simulink model "real_world_idmt_relay_3phase_standalone_2024a"  (R2024a)
settings: Solver=ode23tb  StartTime=0.0  StopTime=10  RelTol=1e-7  EnableMultiTasking=on
libraries: spsThreePhaseVIMeasurementLib x3, spsThreePhaseBreakerLib x2, spsDistributedParametersLineLib x2, spsRMSLib x2, spsThreePhaseFaultLib x2, spsThreePhaseSeriesRLCLoadLib x1, spsThreePhaseSourceLib x1, spspowerguiLib x1
settings Model: Creator=Rodney Tan  LastModifiedBy=user
settings SolverCC: AlgebraicLoopSolver=TrustRegion
settings DataIOCC: LimitDataPoints=on  SaveFormat=Array  ReturnWorkspaceOutputs=off
settings OptimizationCC: LifeSpan=inf
settings DebuggingCC: UnconnectedInputMsg=warning  UnconnectedOutputMsg=warning  UnconnectedLineMsg=warning  SFUnexpectedBacktrackingDiag=warning  SFNoUnconditionalDefaultTransitionDiag=warning  SFExecutionAtInitializationDiag=none  ArithmeticOperatorsInVariantConditions=warning
settings HardwareCC: ProdBitPerPointer=32  ProdBitPerSizeT=32  ProdBitPerPtrDiffT=32  ProdLargestAtomicFloat=None  ProdIntDivRoundTo=Undefined  ProdEndianess=Unspecified  ProdWordSize=32  ProdHWDeviceType=32-bit Generic
settings ModelReferenceCC: EnableRefExpFcnMdlSchedulingChecks=on  PropagateSignalLabelsOutOfModel=off
settings SFSimCC: SimUseLocalCustomCode=off  CustomCodeUndefinedFunction=UseInterfaceOnly
settings RTWCC: RTWUseLocalCustomCode=off  GPUComputeCapability=3.5
settings CodeAppCC: StateflowObjectComments=on
settings GRTTargetCC: TargetLangStandard=C89/C90 (ANSI)
settings ConfigComp: CovMetricSettings=dw  CovSaveCumulativeToWorkspaceVar=on  CovSaveSingleToWorkspaceVar=on  CovExternalEMLEnable=off
settings SimscapeCC: SimscapeNormalizeSystem=off

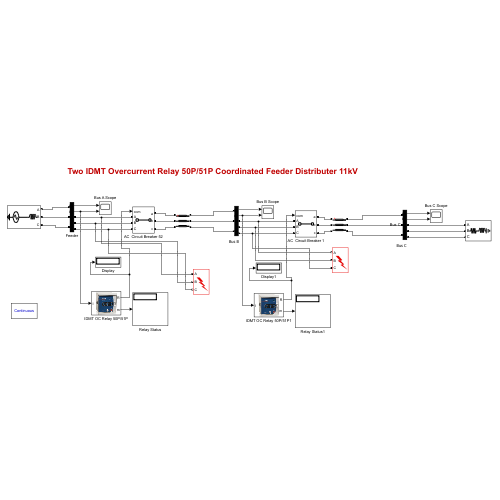
[thumbnail: Simulink's stored preview of the top-level diagram]
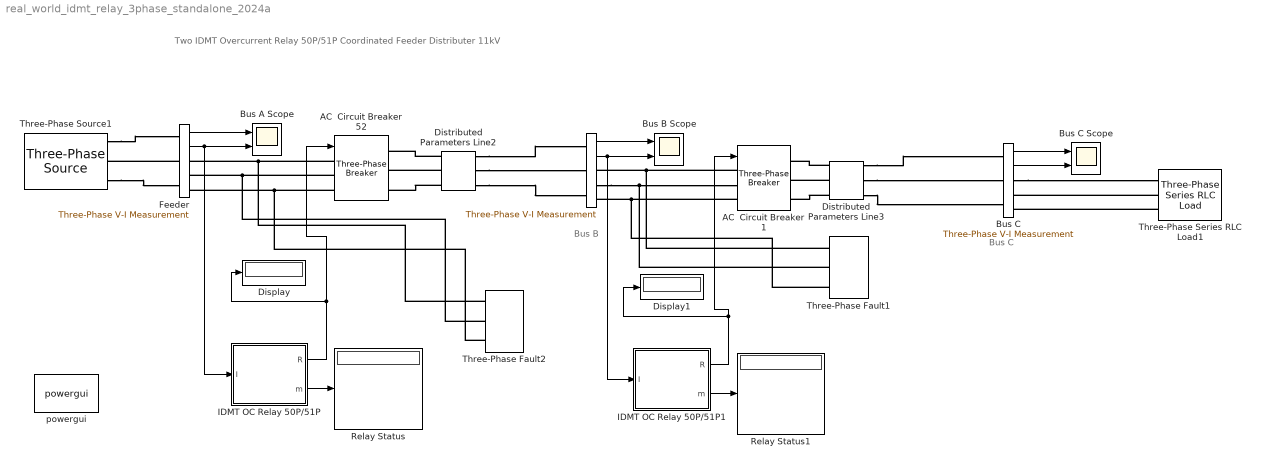
== system real_world_idmt_relay_3phase_standalone_2024a ==
  note: Bus C
  note: Bus B
  note: Two IDMT Overcurrent Relay 50P/51P Coordinated Feeder Distributer 11kV
  " " : spsThreePhaseVIMeasurementLib/Three-Phase V-I Measurement  VoltageMeasurement=phase-to-ground  SetLabelV=off  LabelV=Vabc  Vpu=off  VpuLL=off  CurrentMeasurement=yes  SetLabelI=off  LabelI=Iabc  Ipu=off  Pbase=100e6  Vbase=500e3  OutputType=Complex  PhasorSimulation=off  PSBequivalent=0
  AC  Circuit Breaker 1 : spsThreePhaseBreakerLib/Three-Phase Breaker  InitialState=closed  SwitchA=on  SwitchB=on  SwitchC=on  SwitchTimes="[1/60  5/60]"  External=on  BreakerResistance=0.01  SnubberResistance=1e6  SnubberCapacitance=inf  Measurements=None
  AC  Circuit Breaker 52 : spsThreePhaseBreakerLib/Three-Phase Breaker  InitialState=closed  SwitchA=on  SwitchB=on  SwitchC=on  SwitchTimes="[1/60  5/60]"  External=on  BreakerResistance=0.01  SnubberResistance=1e6  SnubberCapacitance=inf  Measurements=None
  Bus A Scope : Scope  NumInputPorts=2
  Bus B Scope : Scope  NumInputPorts=2
  Bus C : spsThreePhaseVIMeasurementLib/Three-Phase V-I Measurement  VoltageMeasurement=phase-to-ground  SetLabelV=off  LabelV=Vabc  Vpu=off  VpuLL=off  CurrentMeasurement=yes  SetLabelI=off  LabelI=Iabc  Ipu=off  Pbase=100e6  Vbase=500e3  OutputType=Complex  PhasorSimulation=off  PSBequivalent=0
  Bus C Scope : Scope  NumInputPorts=2
  Display : Display
  Display1 : Display
  Distributed Parameters Line2 : spsDistributedParametersLineLib/Distributed Parameters Line  Phases=3  Length=5  Frequency=50  Resistance=[0.306 0.918]  Inductance="[0.2642e-3  1.0504e-3]"  Capacitance=[12.74e-6 7.751e-6]  x1=[3.27922978200512e-12 11154.6811765329 11154.6811765329;314.159265358979 314.159265358979 314.159265358979;-1.12452839492294 0.423971778555255 -1.14682454823964]  x2=[8.7354113531085e-12 10968.40053619 10968.40053619;314.159265358979 314.159265358979 314.159265358979;-0.816475613899162 0.387208845042316 -1.18358748175258]  x3=[1.00471196056486e-12 1773.2701065899 1773.2701065899;314.159265358979 314.159265358979 314.159265358979;-1.33202462135814 0.268764817665929 -1.30203150912897]  x4=[3.36344440757806e-13 2029.84067808505 2029.84067808505;314.159265358979 314.159265358979 314.159265358979;-2.69532472171784 0.432839711669644 -1.13795661512525]  x5=0.000451155472093601  V1=[3.279e-12 1.115e+04 1.115e+04;314.2 314.2 314.2;-1.125 0.424 -1.147]  V2=[8.735e-12 1.097e+04 1.097e+04;314.2 314.2 314.2;-0.8165 0.3872 -1.184]  I1=[1.005e-12 1773 1773;314.2 314.2 314.2;-1.332 0.2688 -1.302]  I2=[3.363e-13 2030 2030;314.2 314.2 314.2;-2.695 0.4328 -1.138]  nHarmo=1  Measurements=None  Decoupling=off  VsMag0=0  VrMag0=0  VsAngle0=0  VrAngle0=0  IsMag0=0  IrMag0=0  IsAngle0=0  IrAngle0=0
      settings: LibrarySourceBlock=sps_lib/Power Grid Elements/Distributed Parameters Line
  Distributed Parameters Line3 : spsDistributedParametersLineLib/Distributed Parameters Line  Phases=3  Length=5  Frequency=50  Resistance=[0.306 0.918]  Inductance="[0.2642e-3  1.0504e-3]"  Capacitance=[12.74e-6 7.751e-6]  x1=[9.97338802310938e-12 10966.6241293561 10966.6241293561;314.159265358979 314.159265358979 314.159265358979;-0.959379717508311 0.387108931168386 -1.18368739562651]  x2=[1.28621974215375e-11 10696.5004802315 10696.5004802315;314.159265358979 314.159265358979 314.159265358979;-0.927132835073057 0.380128350784861 -1.19066797601004]  x3=[1.56443975399813e-12 1729.68176986228 1729.68176986227;314.159265358979 314.159265358979 314.159265358979;-1.2488833894697 0.333543848383118 -1.23725247841178]  x4=[1.04295983599876e-12 1982.49698055263 1982.49698055264;314.159265358979 314.159265358979 314.159265358979;-1.89238449826298 0.33489650149686 -1.23589982529804]  x5=0.000451155472093601  V1=[9.973e-12 1.097e+04 1.097e+04;314.2 314.2 314.2;-0.9594 0.3871 -1.184]  V2=[1.286e-11 1.07e+04 1.07e+04;314.2 314.2 314.2;-0.9271 0.3801 -1.191]  I1=[1.564e-12 1730 1730;314.2 314.2 314.2;-1.249 0.3335 -1.237]  I2=[1.043e-12 1982 1982;314.2 314.2 314.2;-1.892 0.3349 -1.236]  nHarmo=1  Measurements=None  Decoupling=off  VsMag0=0  VrMag0=0  VsAngle0=0  VrAngle0=0  IsMag0=0  IrMag0=0  IsAngle0=0  IrAngle0=0
      settings: LibrarySourceBlock=sps_lib/Power Grid Elements/Distributed Parameters Line
  Feeder : spsThreePhaseVIMeasurementLib/Three-Phase V-I Measurement  VoltageMeasurement=phase-to-ground  SetLabelV=off  LabelV=Vabc  Vpu=off  VpuLL=off  CurrentMeasurement=yes  SetLabelI=off  LabelI=Iabc  Ipu=off  Pbase=100e6  Vbase=500e3  OutputType=Complex  PhasorSimulation=off  PSBequivalent=0
  IDMT OC Relay 50P/51P : Subsystem  mask(IDMT Overcurrent Relay 50P/51P Block){Lowset_idx=5, TMS_idx=0.2, Highset_idx=x10, CTpri=400, Freq=50}
      mask prompts: Lowset_idx "Low-set (I>)"; TMS_idx "TMS"; Highset_idx "High-set (I>>)"; CTpri "CT Primary (A) / 5A"; Freq "Fundamental frequency (Hz):"
      mask help:
      | IDMT Overcurrent Relay 50P/51P Block developed by Dr Rodney Tan
      | Version 1.0 (Apr 2021)
      |
      | This relay block combine IDMT Overcurrent Relay and Instantaneous Relay (ANSI/IEEE C37.2 device number 50P and 51P) that operates when the current exceeds a predetermined value.
      |
      | Relay 51P operates based on IEC 60255 Standard Normal Inverse IDMT (Inverse Definite Minimum Time) trip characteristic.
      mask Help:
      | <b><u>Block Setting</u></b>
      | 
      | <b>Low-set (I >)</b>
      | Specify relay pick-up current based on current transformer rating ranging from 2A to 6A (40%-120%).
      | 
      | <b>Time Multiplier Setting (TMS)</b>
      | Specify time delay multiplier ranging from 0.05 to 1.0 for IDMT relay operation.
      | 
      | <b>Current Transformer Primary (A)</b>
      | Specify current transformer primary in Ampere.
      | 
      | <b>Fundamental Frequency (Hz)</b>
      | Specify the RMS current measurement fundamental frequency, in hertz, of the input signal.
      | 
      | <b>Plot IDMT IEC Normal Inverse Curve Button</b>
      | Plot IDMT IEC Normal Inverse curve with all TM.
      | 
      | <b><u>Block Input Output</u></b>
      | <b>I</b>
      | Current input to the overcurrent relay
      | 
      | <b>R</b>
      | Relay output (1-0) control signal, commonly connected to circuit breaker
      | 
      | <b>m</b>
      | Relay operating time, CT Primary current, CT secondary current and PSM
      mask TypeOptions Lowset_idx: 2 | 2.5 | 3 | 3.5 | 4 | 4.5 | 5 | 5.5 | 6
      mask TypeOptions TMS_idx: 0.05 | 0.1 | 0.2 | 0.3 | 0.4 | 0.5 | 0.6 | 0.7 | 0.8 | 0.9 | 1.0
      mask TypeOptions Highset_idx: x1 | x2 | x3 | x4 | x5 | x6 | x7 | x8 | x9 | x10 | inf
      mask TypeOptions Freq: Irms/Freq
      mask DialogControl Container6 Prompt: Relay Setting
      mask DialogControl Container7 Prompt: Current Transformer Setting
      mask DialogControl plotbutton Prompt: Plot IDMT IEC Normal Inverse Curve
      mask DialogControl plotbutton Callback:
      | % Plotting IDMT Curve
      | TMS = str2double(get_param(gcb,'TMS_idx'));
      | I = 1:20;
      | IDMTCurve = (3./log10(I))*0.05;
      | if TMS == 0.05
      |     loglog(IDMTCurve,'color','r','linewidth',2);
      | else
      |     loglog(IDMTCurve,'color','b');
      | end
      | hold on
      | for nTMS = 1:10
      |     IDMTCurve = (3./log10(I))*nTMS*0.1;
      |     if round(nTMS*0.1,1) == TMS
      |         loglog(IDMTCurve,'color','r','linewidth',2);
      |     else
      |         loglog(IDMTCurve,'color','b');
      |     end
      | end
      | hold off
      | set(gcf, 'Position', [200 150 300 500]);
      | title('IEC Normal Inverse Curve');
      | xlim([1 30]);
      | set(gca, 'XTick', [1:10 20]);
      | ylim([0.1 10]);
      | set(gca, 'YTick', [0.1 1:10]);
      | yticklabels([0.1 1:10]);
      | xlabel('Current (Multiples of Plug Setting)');
      | ylabel('Operating Time (sec)');
      | grid on;
      mask Display: image('$imagefile'); % Use "Edit Image" on toolstrip to change.
  IDMT OC Relay 50P/51P1 : Subsystem  mask(IDMT Overcurrent Relay 50P/51P Block){Lowset_idx=3.5, TMS_idx=0.2, Highset_idx=x10, CTpri=300, Freq=50}
      mask prompts: Lowset_idx "Low-set (I>)"; TMS_idx "TMS"; Highset_idx "High-set (I>>)"; CTpri "CT Primary (A) / 5A"; Freq "Fundamental frequency (Hz):"
      mask help:
      | IDMT Overcurrent Relay 50P/51P Block developed by Dr Rodney Tan
      | Version 1.0 (Apr 2021)
      |
      | This relay block combine IDMT Overcurrent Relay and Instantaneous Relay (ANSI/IEEE C37.2 device number 50P and 51P) that operates when the current exceeds a predetermined value.
      |
      | Relay 51P operates based on IEC 60255 Standard Normal Inverse IDMT (Inverse Definite Minimum Time) trip characteristic.
      mask Help:
      | <b><u>Block Setting</u></b>
      | 
      | <b>Low-set (I >)</b>
      | Specify relay pick-up current based on current transformer rating ranging from 2A to 6A (40%-120%).
      | 
      | <b>Time Multiplier Setting (TMS)</b>
      | Specify time delay multiplier ranging from 0.05 to 1.0 for IDMT relay operation.
      | 
      | <b>Current Transformer Primary (A)</b>
      | Specify current transformer primary in Ampere.
      | 
      | <b>Fundamental Frequency (Hz)</b>
      | Specify the RMS current measurement fundamental frequency, in hertz, of the input signal.
      | 
      | <b>Plot IDMT IEC Normal Inverse Curve Button</b>
      | Plot IDMT IEC Normal Inverse curve with all TM.
      | 
      | <b><u>Block Input Output</u></b>
      | <b>I</b>
      | Current input to the overcurrent relay
      | 
      | <b>R</b>
      | Relay output (1-0) control signal, commonly connected to circuit breaker
      | 
      | <b>m</b>
      | Relay operating time, CT Primary current, CT secondary current and PSM
      mask TypeOptions Lowset_idx: 2 | 2.5 | 3 | 3.5 | 4 | 4.5 | 5 | 5.5 | 6
      mask TypeOptions TMS_idx: 0.05 | 0.1 | 0.2 | 0.3 | 0.4 | 0.5 | 0.6 | 0.7 | 0.8 | 0.9 | 1.0
      mask TypeOptions Highset_idx: x1 | x2 | x3 | x4 | x5 | x6 | x7 | x8 | x9 | x10 | inf
      mask TypeOptions Freq: Irms/Freq
      mask DialogControl Container6 Prompt: Relay Setting
      mask DialogControl Container7 Prompt: Current Transformer Setting
      mask DialogControl plotbutton Prompt: Plot IDMT IEC Normal Inverse Curve
      mask DialogControl plotbutton Callback:
      | % Plotting IDMT Curve
      | TMS = str2double(get_param(gcb,'TMS_idx'));
      | I = 1:20;
      | IDMTCurve = (3./log10(I))*0.05;
      | if TMS == 0.05
      |     loglog(IDMTCurve,'color','r','linewidth',2);
      | else
      |     loglog(IDMTCurve,'color','b');
      | end
      | hold on
      | for nTMS = 1:10
      |     IDMTCurve = (3./log10(I))*nTMS*0.1;
      |     if round(nTMS*0.1,1) == TMS
      |         loglog(IDMTCurve,'color','r','linewidth',2);
      |     else
      |         loglog(IDMTCurve,'color','b');
      |     end
      | end
      | hold off
      | set(gcf, 'Position', [200 150 300 500]);
      | title('IEC Normal Inverse Curve');
      | xlim([1 30]);
      | set(gca, 'XTick', [1:10 20]);
      | ylim([0.1 10]);
      | set(gca, 'YTick', [0.1 1:10]);
      | yticklabels([0.1 1:10]);
      | xlabel('Current (Multiples of Plug Setting)');
      | ylabel('Operating Time (sec)');
      | grid on;
      mask Display: image('OCRelayIcon_1.jpg');
  Relay Status : Display
  Relay Status1 : Display
  Three-Phase Series RLC Load1 : spsThreePhaseSeriesRLCLoadLib/Three-Phase Series RLC Load  LConnTagsString=A|B|C  Configuration=Y (grounded)  NominalVoltage=11000  Vabc=[1e3 1e3 1e3]  Vabcp=[1e3 1e3 1e3]  NominalFrequency=50  UnbalancedPower=off  ActivePower=2e6  InductivePower=1.2e6  CapacitivePower=0  Pabc=[10e3 9e3 11e3]  QLabc=[100 90 110]  QCabc=[100 90 110]  Pabcp=[10e3 9e3 11e3]  QLabcp=[100 90 110]  QCabcp=[100 90 110]  Measurements=None  LoadType=constant Z
  Three-Phase Fault1 : spsThreePhaseFaultLib/Three-Phase Fault  InitialStates=0  FaultA=off  FaultB=off  FaultC=off  GroundFault=off  SwitchTimes=[0.2 0.5]  External=off  SwitchStatus=NaN  FaultResistance=0.01  GroundResistance=0.01  SnubberResistance=1e6  SnubberCapacitance=inf  Measurements=None
  Three-Phase Fault2 : spsThreePhaseFaultLib/Three-Phase Fault  InitialStates=0  FaultA=off  FaultB=on  FaultC=off  GroundFault=on  SwitchTimes=[0.2 0.5]  External=off  SwitchStatus=NaN  FaultResistance=0.01  GroundResistance=0.01  SnubberResistance=1e6  SnubberCapacitance=inf  Measurements=None
  Three-Phase Source1 : spsThreePhaseSourceLib/Three-Phase Source  InternalConnection=Yg  VoltagePhases=off  Voltage=11000  PhaseAngle=0  Voltage_phases=[25e3 25e3 25e3]/sqrt(3)  PhaseAngles_phases=[0 -120 +120]  Frequency=50  NonIdealSource=on  SpecifyImpedance=off  Resistance=0.0  Inductance=1.540e-3  ShortCircuitLevel=100e6  BaseVoltage=11000  XRratio=7  BusType=swing  Pref=10e3  Qref=0  Prefabc=[10e3, 10e3, 10e3]  Qrefabc=[0, 0, 0]  Qmin=-inf  Qmax=inf
  powergui : spspowerguiLib/powergui  Priority=1  SimulationMode=Continuous  SampleTime=50e-6  frequency=60  Iterations=50  frequencyindice=50  Pbase=100e6  ErrMax=1e-4  UnitsV=kV  UnitsW=MW  buscounter=0  FunctionMessages=off  echomessages=off  EnableUseOfTLC=off  CurrentSourceSwitches=off  DisableSnubberDevices=on  DisableRonSwitches=off  DisableVfSwitches=off  DisplayEquations=off  AutomaticDiscreteSolvers=off  SolverType=Tustin/Backward Euler (TBE)  Interpol=off  ExternalGateDelay=off  methode=off  Ts=100  x0status=blocks  SPID=on  SwTol=0  HookPort=off  NonlinearTolerance=1e-4  nMaxIteration=100  ContinueOnMaxIteration=off  RestoreLinks=warning  ResistiveCurrentMeasurement=off  Frange=[0:2:500]  Ylog=off  Xlog=on  ShowGrid=off  save=off  variable=ZData  structure=0  ZoomFFT=off  StartTime=0.0  cycles=1  DisplayStyle=1  fundamental=60  FreqAxis=off  MaxFrequency=1000  frequencyindicesteady=1  RmsSteady=1  display=off
  wires:
  Feeder/2 -> IDMT OC Relay 50P/51P/1(I), Bus A Scope/2
  IDMT OC Relay 50P/51P/1(R) -> AC  Circuit Breaker 52/1, Display/1
  Feeder/1 -> Bus A Scope/1
  IDMT OC Relay 50P/51P/2(m) -> Relay Status/1
  " "/1 -> Bus B Scope/1
  " "/2 -> IDMT OC Relay 50P/51P1/1(I), Bus B Scope/2
  IDMT OC Relay 50P/51P1/2(m) -> Relay Status1/1
  IDMT OC Relay 50P/51P1/1(R) -> AC  Circuit Breaker 1/1, Display1/1
  Bus C/1 -> Bus C Scope/1
  Bus C/2 -> Bus C Scope/2
  connections:
  Three-Phase Source1/RConn1 -- Feeder/LConn1
  AC  Circuit Breaker 52/LConn2 -- Three-Phase Fault2/LConn2 -- Feeder/RConn2
  AC  Circuit Breaker 52/LConn1 -- Three-Phase Fault2/LConn1 -- Feeder/RConn1
  Three-Phase Source1/RConn3 -- Feeder/LConn3
  AC  Circuit Breaker 52/LConn3 -- Three-Phase Fault2/LConn3 -- Feeder/RConn3
  Distributed Parameters Line2/RConn2 -- " "/LConn2
  Feeder/LConn2 -- Three-Phase Source1/RConn2
  Distributed Parameters Line3/RConn2 -- Bus C/LConn2
  Distributed Parameters Line3/RConn3 -- Bus C/LConn3
  Distributed Parameters Line3/LConn1 -- AC  Circuit Breaker 1/RConn1
  Distributed Parameters Line3/RConn1 -- Bus C/LConn1
  Distributed Parameters Line2/LConn2 -- AC  Circuit Breaker 52/RConn2
  Distributed Parameters Line2/LConn3 -- AC  Circuit Breaker 52/RConn3
  Distributed Parameters Line2/LConn1 -- AC  Circuit Breaker 52/RConn1
  Distributed Parameters Line2/RConn3 -- " "/LConn3
  Distributed Parameters Line2/RConn1 -- " "/LConn1
  Distributed Parameters Line3/LConn2 -- AC  Circuit Breaker 1/RConn2
  Distributed Parameters Line3/LConn3 -- AC  Circuit Breaker 1/RConn3
  AC  Circuit Breaker 1/LConn1 -- Three-Phase Fault1/LConn1 -- " "/RConn1
  " "/RConn2 -- Three-Phase Fault1/LConn2 -- AC  Circuit Breaker 1/LConn2
  AC  Circuit Breaker 1/LConn3 -- Three-Phase Fault1/LConn3 -- " "/RConn3
  Three-Phase Series RLC Load1/LConn2 -- Bus C/RConn2
  Three-Phase Series RLC Load1/LConn3 -- Bus C/RConn3
  Bus C/RConn1 -- Three-Phase Series RLC Load1/LConn1

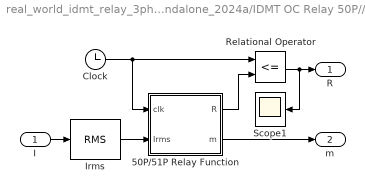
== system real_world_idmt_relay_3phase_standalone_2024a/IDMT OC Relay 50P//51P ==
  I : Inport
  50P/51P Relay Function : MATLAB Function  TreatAsAtomicUnit=on
  Clock : Clock
  Irms : spsRMSLib/RMS  TrueRMS=on  Freq=Freq  RMSInit=0  Ts=0
  Relational Operator : RelationalOperator  Operator=<=  OutDataTypeStr=boolean  InputSameDT=off
  Scope1 : Scope
  R : Outport  VectorParamsAs1DForOutWhenUnconnected=off
  m : Outport  Port=2  VectorParamsAs1DForOutWhenUnconnected=off
  wires:
  Clock/1 -> Relational Operator/1, 50P/51P Relay Function/1(clk)
  Irms/1 -> 50P/51P Relay Function/2(Irms)
  50P/51P Relay Function/1(R) -> Relational Operator/2
  Relational Operator/1 -> Scope1/1, R/1
  I/1 -> Irms/1
  50P/51P Relay Function/2(m) -> m/1

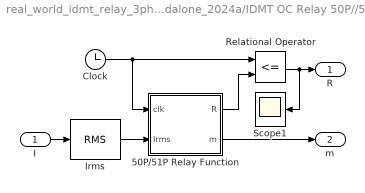
== system real_world_idmt_relay_3phase_standalone_2024a/IDMT OC Relay 50P//51P1 ==
  I : Inport
  50P/51P Relay Function : MATLAB Function  TreatAsAtomicUnit=on
  Clock : Clock
  Irms : spsRMSLib/RMS  TrueRMS=on  Freq=Freq  RMSInit=0  Ts=0
  Relational Operator : RelationalOperator  Operator=<=  OutDataTypeStr=boolean  InputSameDT=off
  Scope1 : Scope
  R : Outport  VectorParamsAs1DForOutWhenUnconnected=off
  m : Outport  Port=2  VectorParamsAs1DForOutWhenUnconnected=off
  wires:
  Clock/1 -> Relational Operator/1, 50P/51P Relay Function/1(clk)
  Irms/1 -> 50P/51P Relay Function/2(Irms)
  50P/51P Relay Function/1(R) -> Relational Operator/2
  Relational Operator/1 -> Scope1/1, R/1
  I/1 -> Irms/1
  50P/51P Relay Function/2(m) -> m/1

== matlab function real_world_idmt_relay_3phase_standalone_2024a/IDMT OC Relay 50P//51P/50P//51P Relay Function ==
  settings: updateMethod=DISCRETE
  data: R output; clk input; Irms input; CTpri parameter; Lowset_idx parameter; m output; TMS_idx parameter; Highset_idx parameter
function [R, m] = fcn(clk,Irms,CTpri,Lowset_idx,TMS_idx,Highset_idx)

persistent RelayState TripTime OperatingTime PickupTime mFaultPri mFaultSec PSM

if isempty(RelayState)
    RelayState = 0;
    TripTime = inf;
    OperatingTime = inf;
    PickupTime = 0;
    mFaultPri = 0;
    mFaultSec = 0;
    PSM = 0;
end

Lowset = [2 2.5 3 3.5 4 4.5 5 5.5 6];
TMS = [0.05 0.1 0.2 0.3 0.4 0.5 0.6 0.7 0.8 0.9 1.0];
Highset = [1 2 3 4 5 6 7 8 9 10 Inf];

FaultSec = max(Irms/(CTpri/5));
FaultPri = max(Irms);
Pickup = Lowset(Lowset_idx); % CT secondary pick up

% Record highest fault current
if FaultPri > mFaultPri
    mFaultPri = FaultPri;
    mFaultSec = FaultSec;
end

if (RelayState == 0)&&(FaultSec > Pickup)
    PickupTime = clk;
    RelayState = 1;
end

if (RelayState == 1)&&(clk>(PickupTime+0.02)) % Wait for 20ms fault current rise time

    PSM = FaultSec/Pickup;   % Calculate Plug Multiplier Setting
    
    if PSM <= Highset(Highset_idx)
        if PSM <= 20
            OperatingTime = (3/log10(PSM))*TMS(TMS_idx);
        else
            OperatingTime = (3/log10(20))*TMS(TMS_idx);
        end
    else
        OperatingTime = 0.04;
    end
    TripTime = PickupTime + OperatingTime;
    RelayState = 2;
end

% Resetting Relay
if (RelayState == 2)&&(FaultSec < Pickup)
    OperatingTime = inf;
    TripTime = inf;
    RelayState = 0;
end

if(clk>TripTime)
    RelayState=-1;
end

R = TripTime;
m = [OperatingTime mFaultPri mFaultSec PSM];

== matlab function real_world_idmt_relay_3phase_standalone_2024a/IDMT OC Relay 50P//51P1/50P//51P Relay Function ==
  settings: updateMethod=DISCRETE
  data: R output; clk input; Irms input; CTpri parameter; Lowset_idx parameter; m output; TMS_idx parameter; Highset_idx parameter
function [R, m] = fcn(clk,Irms,CTpri,Lowset_idx,TMS_idx,Highset_idx)

persistent RelayState TripTime OperatingTime PickupTime mFaultPri mFaultSec PSM

if isempty(RelayState)
    RelayState = 0;
    TripTime = inf;
    OperatingTime = inf;
    PickupTime = 0;
    mFaultPri = 0;
    mFaultSec = 0;
    PSM = 0;
end

Lowset = [2 2.5 3 3.5 4 4.5 5 5.5 6];
TMS = [0.05 0.1 0.2 0.3 0.4 0.5 0.6 0.7 0.8 0.9 1.0];
Highset = [1 2 3 4 5 6 7 8 9 10 Inf];

FaultSec = max(Irms/(CTpri/5));
FaultPri = max(Irms);
Pickup = Lowset(Lowset_idx); % CT secondary pick up

% Record highest fault current
if FaultPri > mFaultPri
    mFaultPri = FaultPri;
    mFaultSec = FaultSec;
end

if (RelayState == 0)&&(FaultSec > Pickup)
    PickupTime = clk;
    RelayState = 1;
end

if (RelayState == 1)&&(clk>(PickupTime+0.02)) % Wait for 20ms fault current rise time

    PSM = FaultSec/Pickup;   % Calculate Plug Multiplier Setting
    
    if PSM <= Highset(Highset_idx)
        if PSM <= 20
            OperatingTime = (3/log10(PSM))*TMS(TMS_idx);
        else
            OperatingTime = (3/log10(20))*TMS(TMS_idx);
        end
    else
        OperatingTime = 0.04;
    end
    TripTime = PickupTime + OperatingTime;
    RelayState = 2;
end

% Resetting Relay
if (RelayState == 2)&&(FaultSec < Pickup)
    OperatingTime = inf;
    TripTime = inf;
    RelayState = 0;
end

if(clk>TripTime)
    RelayState=-1;
end

R = TripTime;
m = [OperatingTime mFaultPri mFaultSec PSM];
